simulink model "simulated_system_LQR"  (R2026a)
settings: Solver=ode4  StopTime=Tsim  FixedStep=h
undefined symbols (not defined in the file or in its folder): K, x0
settings Model: Creator=luca  LastModifiedBy=luca

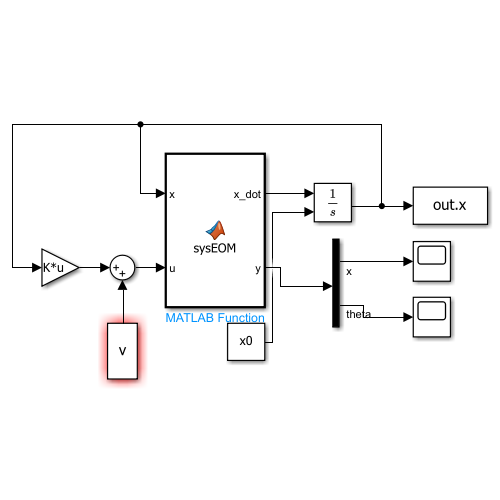
[thumbnail: Simulink's stored preview of the top-level diagram]
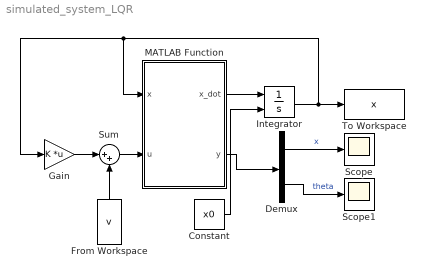
== system simulated_system_LQR ==
  Constant : Constant  Value=x0
  Demux : Demux  Outputs=2
  From Workspace : FromWorkspace  VariableName=v
  Gain : Gain  Gain=K  Multiplication=Matrix(K*u)
  Integrator : Integrator  InitialConditionSource=external  InitialCondition=[0;0;0;0]
  MATLAB Function : MATLAB Function  TreatAsAtomicUnit=on
  Scope : Scope
  Scope1 : Scope
  Sum : Sum  Inputs=|++
  To Workspace : ToWorkspace  VariableName=x  SampleTime=-1
  wires:
  Demux/2 -> Scope1/1  "theta"
  Demux/1 -> Scope/1  "x"
  Integrator/1 -> Gain/1, MATLAB Function/1(x), To Workspace/1
  MATLAB Function/2(y) -> Demux/1
  MATLAB Function/1(x_dot) -> Integrator/1
  Constant/1 -> Integrator/2
  Gain/1 -> Sum/1
  Sum/1 -> MATLAB Function/2(u)
  From Workspace/1 -> Sum/2

== matlab function simulated_system_LQR/MATLAB Function ==
  data: x input size=4; x_dot output size=4; u input size=1; y output size=2; param parameter
function [x_dot, y] = sysEOM(x, u, param)
% x = [x, v, \theta, \omega]
% y = sensor data (position and angle)

M   = param.M;
m   = param.m;
g   = param.g;
b   = param.b;
c   = param.c;
l   = param.l;
k_m = param.k_m;

f = k_m * u;
D      = (M + m)*m*l^2 - (m*l*cos(x(3)))^2;
phi    = f - c*x(2) + m*l*x(4)^2*sin(x(3));
psi    = m*g*l*sin(x(3)) - b*x(4);

x_dot    = zeros(4,1);
x_dot(1) = x(2);
x_dot(2) = ( m*l^2 * phi  -  m*l*cos(x(3)) * psi ) / D;
x_dot(3) = x(4);
x_dot(4) = ( (M+m) * psi  -  m*l*cos(x(3)) * phi ) / D;

y = [x(1), x(3)]';
end
